simulink model "LowPassFilter"  (R2021b)
settings: Solver=VariableStepAuto  StartTime=0.0  StopTime=1  RelTol=1e-3
libraries: simulink x1
settings Model: Creator=win  LastModifiedBy=win

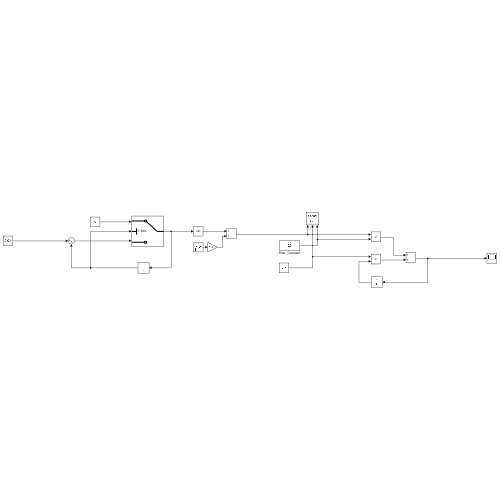
[thumbnail: Simulink's stored preview of the top-level diagram]
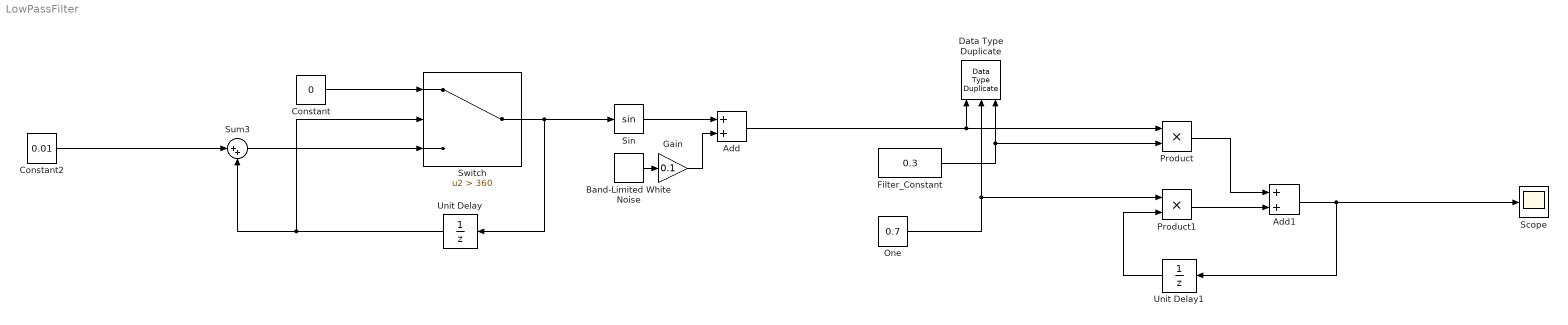
== system LowPassFilter ==
  Add : Sum
  Add1 : Sum  RndMeth=Simplest  OutDataTypeStr=Inherit: Same as first input
  Band-Limited White Noise : simulink/Sources/Band-Limited White Noise  Cov=[0.001]  Ts=0.001  seed=[111111]
  Constant : Constant  Value=0
  Constant2 : Constant  Value=0.01
  Data Type Duplicate : DataTypeDuplicate  NumInputPorts=3
  Filter_Constant : Constant  Value=0.3  OutDataTypeStr=Inherit: Inherit via back propagation
  Gain : Gain  Gain=0.1
  One : Constant  Value=0.7  OutDataTypeStr=Inherit: Inherit via back propagation
  Product : Product  RndMeth=Simplest  OutDataTypeStr=Inherit: Same as first input
  Product1 : Product  RndMeth=Simplest  OutDataTypeStr=Inherit: Same as first input
  Scope : Scope
  Sin : Trigonometry
  Sum3 : Sum  Inputs=|++
  Switch : Switch  Criteria=u2 > Threshold  Threshold=360
  Unit Delay : UnitDelay  SampleTime=0.001  HasFrameUpgradeWarning=on
  Unit Delay1 : UnitDelay  SampleTime=0.001  HasFrameUpgradeWarning=on
  wires:
  Constant2/1 -> Sum3/1
  Switch/1 -> Unit Delay/1, Sin/1
  Sum3/1 -> Switch/3
  Unit Delay/1 -> Switch/2, Sum3/2
  Constant/1 -> Switch/1
  Sin/1 -> Add/1
  Add/1 -> Data Type Duplicate/1, Product/1
  Filter_Constant/1 -> Product/2, Data Type Duplicate/3
  One/1 -> Data Type Duplicate/2, Product1/1
  Add1/1 -> Unit Delay1/1, Scope/1
  Unit Delay1/1 -> Product1/2
  Product1/1 -> Add1/2
  Product/1 -> Add1/1
  Band-Limited White Noise/1 -> Gain/1
  Gain/1 -> Add/2
